simulink library "fixpt_dtprop"  (Simulink 5.0)
undefined symbols (not defined in the file or in its folder): Bias1, Bias2, NumBits1, NumBits2, PosRange1, PosRange2, Slope1, Slope2
libraries: fixpt3 x29, fixpt_lib_4 x1
settings Model: Creator=andyb  LastModifiedBy=kgondoly  ExtModeAutoUpdateStatusClock=off

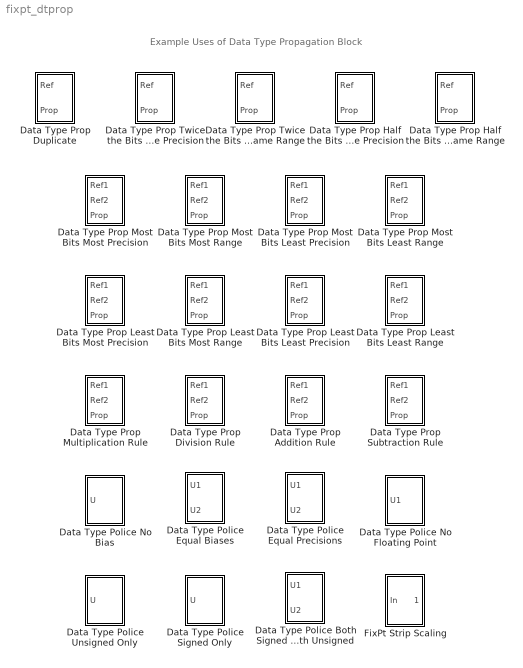
== system fixpt_dtprop ==
  note: Example Uses of Data Type Propagation Block
  Data Type Police Both Signed or Both Unsigned : Subsystem
  Data Type Police Equal Biases : Subsystem
  Data Type Police Equal Precisions : Subsystem
  Data Type Police No Bias : Subsystem
  Data Type Police No Floating Point : Subsystem
  Data Type Police Signed Only : Subsystem
  Data Type Police Unsigned Only : Subsystem
  Data Type Prop Addition Rule : Subsystem
  Data Type Prop Division Rule : Subsystem
  Data Type Prop Duplicate : Subsystem
  Data Type Prop Half the Bits Same Precision : Subsystem
  Data Type Prop Half the Bits Same Range : Subsystem
  Data Type Prop Least Bits Least Precision : Subsystem
  Data Type Prop Least Bits Least Range : Subsystem
  Data Type Prop Least Bits Most Precision : Subsystem
  Data Type Prop Least Bits Most Range : Subsystem
  Data Type Prop Most Bits Least Precision : Subsystem
  Data Type Prop Most Bits Least Range : Subsystem
  Data Type Prop Most Bits Most Precision : Subsystem
  Data Type Prop Most Bits Most Range : Subsystem
  Data Type Prop Multiplication Rule : Subsystem
  Data Type Prop Subtraction Rule : Subsystem
  Data Type Prop Twice the Bits Same Precision : Subsystem
  Data Type Prop Twice the Bits Same Range : Subsystem
  FixPt Strip Scaling : Subsystem
      mask Type: Fixed-Point Strip Scaling
      mask Description: This block strips the scaling off a fixed point signal.  It maps the input data type to the smallest builtin data type that has sufficient bits to hold the input.  The stored Integer Value of the input will be the value of the output.  The output always has nominal scaling (slope = 1.0 and bias = 0.0), so the output does not have a distinction between Real World Value and Stored Integer Value.
      mask Display: fprintf('Strip')

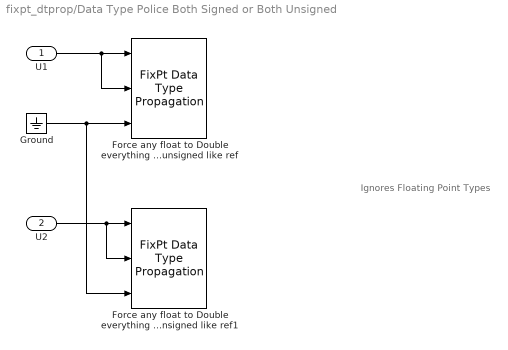
== system fixpt_dtprop/Data Type Police Both Signed or Both Unsigned ==
  note: Ignores Floating Point Types
  U1 : Inport
  U2 : Inport  Port=2
  Force any float to Double everything else to 8 bits with nominal scaling but signed or unsigned like ref : fixpt3/FixPt Data Type Propagation  PropDataType=ufix(8)  IfRefDouble=double  IfRefSingle=double  IsSigned=IsSigned1  NumBitsBase=NumBits1  NumBitsMult=0  NumBitsAdd=8  NumBitsAllowFinal=1:128  PropScalingMode=Specify via dialog  PropScaling=1  SlopeBase=Slope1  SlopeMult=0  SlopeAdd=1  BiasBase=Bias1  BiasMult=1  BiasAdd=0
  Force any float to Double everything else to 8 bits with nominal scaling but signed or unsigned like ref1 : fixpt3/FixPt Data Type Propagation  PropDataType=ufix(8)  IfRefDouble=double  IfRefSingle=double  IsSigned=IsSigned1  NumBitsBase=NumBits1  NumBitsMult=0  NumBitsAdd=8  NumBitsAllowFinal=1:128  PropScalingMode=Specify via dialog  PropScaling=1  SlopeBase=Slope1  SlopeMult=0  SlopeAdd=1  BiasBase=Bias1  BiasMult=1  BiasAdd=0
  Ground : Ground
  wires:
  U1/1 -> Force any float to Double everything else to 8 bits with nominal scaling but signed or unsigned like ref/1, Force any float to Double everything else to 8 bits with nominal scaling but signed or unsigned like ref/2
  Ground/1 -> Force any float to Double everything else to 8 bits with nominal scaling but signed or unsigned like ref1/3, Force any float to Double everything else to 8 bits with nominal scaling but signed or unsigned like ref/3
  U2/1 -> Force any float to Double everything else to 8 bits with nominal scaling but signed or unsigned like ref1/2, Force any float to Double everything else to 8 bits with nominal scaling but signed or unsigned like ref1/1

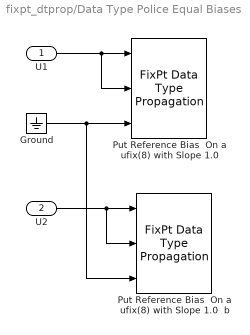
== system fixpt_dtprop/Data Type Police Equal Biases ==
  U1 : Inport
  U2 : Inport  Port=2
  Ground : Ground
  Put Reference Bias  On a ufix(8) with Slope 1.0 : fixpt3/FixPt Data Type Propagation  PropDataTypeMode=Specify via dialog  PropDataType=ufix(8)  IfRefDouble=double  IfRefSingle=double  IsSigned=IsSigned1  NumBitsBase=NumBits1  NumBitsMult=1  NumBitsAdd=0  NumBitsAllowFinal=1:128  PropScaling=2^-10  SlopeBase=Slope1  SlopeMult=0  SlopeAdd=1  BiasBase=Bias1  BiasMult=1  BiasAdd=0
  Put Reference Bias  On a ufix(8) with Slope 1.0  b : fixpt3/FixPt Data Type Propagation  PropDataTypeMode=Specify via dialog  PropDataType=ufix(8)  IfRefDouble=double  IfRefSingle=double  IsSigned=IsSigned1  NumBitsBase=NumBits1  NumBitsMult=1  NumBitsAdd=0  NumBitsAllowFinal=1:128  PropScaling=2^-10  SlopeBase=Slope1  SlopeMult=0  SlopeAdd=1  BiasBase=Bias1  BiasMult=1  BiasAdd=0
  wires:
  U1/1 -> Put Reference Bias  On a ufix(8) with Slope 1.0/2, Put Reference Bias  On a ufix(8) with Slope 1.0/1
  Ground/1 -> Put Reference Bias  On a ufix(8) with Slope 1.0  b/3, Put Reference Bias  On a ufix(8) with Slope 1.0/3
  U2/1 -> Put Reference Bias  On a ufix(8) with Slope 1.0  b/2, Put Reference Bias  On a ufix(8) with Slope 1.0  b/1

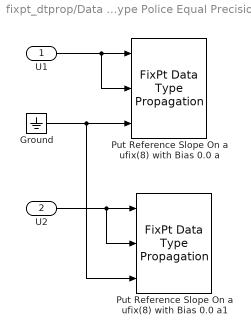
== system fixpt_dtprop/Data Type Police Equal Precisions ==
  U1 : Inport
  U2 : Inport  Port=2
  Ground : Ground
  Put Reference Slope On a ufix(8) with Bias 0.0 a : fixpt3/FixPt Data Type Propagation  PropDataTypeMode=Specify via dialog  PropDataType=ufix(8)  IfRefDouble=double  IfRefSingle=double  IsSigned=IsSigned1  NumBitsBase=NumBits1  NumBitsMult=1  NumBitsAdd=0  NumBitsAllowFinal=1:128  PropScaling=2^-10  SlopeBase=Slope1  SlopeMult=1  SlopeAdd=0  BiasBase=Bias1  BiasMult=0  BiasAdd=0
  Put Reference Slope On a ufix(8) with Bias 0.0 a1 : fixpt3/FixPt Data Type Propagation  PropDataTypeMode=Specify via dialog  PropDataType=ufix(8)  IfRefDouble=double  IfRefSingle=double  IsSigned=IsSigned1  NumBitsBase=NumBits1  NumBitsMult=1  NumBitsAdd=0  NumBitsAllowFinal=1:128  PropScaling=2^-10  SlopeBase=Slope1  SlopeMult=1  SlopeAdd=0  BiasBase=Bias1  BiasMult=0  BiasAdd=0
  wires:
  U2/1 -> Put Reference Slope On a ufix(8) with Bias 0.0 a1/1, Put Reference Slope On a ufix(8) with Bias 0.0 a1/2
  Ground/1 -> Put Reference Slope On a ufix(8) with Bias 0.0 a/3, Put Reference Slope On a ufix(8) with Bias 0.0 a1/3
  U1/1 -> Put Reference Slope On a ufix(8) with Bias 0.0 a/1, Put Reference Slope On a ufix(8) with Bias 0.0 a/2

== system fixpt_dtprop/Data Type Police No Bias ==
  U : Inport
  FixPt Data Type Propagation : fixpt3/FixPt Data Type Propagation  PropDataType=sfix(16)  IfRefDouble=double  IfRefSingle=single  IsSigned=IsSigned1  NumBitsBase=NumBits1  NumBitsMult=1  NumBitsAdd=0  NumBitsAllowFinal=1:128  PropScaling=2^-10  SlopeBase=Slope1  SlopeMult=1  SlopeAdd=0  BiasBase=Bias1  BiasMult=0  BiasAdd=0
  wires:
  U/1 -> FixPt Data Type Propagation/3, FixPt Data Type Propagation/2, FixPt Data Type Propagation/1

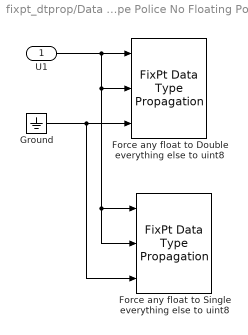
== system fixpt_dtprop/Data Type Police No Floating Point ==
  U1 : Inport
  Force any float to Double everything else to uint8 : fixpt3/FixPt Data Type Propagation  PropDataType=ufix(8)  IfRefDouble=double  IfRefSingle=double  IsSigned=FALSE  NumBitsBase=NumBits1  NumBitsMult=0  NumBitsAdd=8  NumBitsAllowFinal=1:128  PropScalingMode=Specify via dialog  PropScaling=1  SlopeBase=Slope1  SlopeMult=0  SlopeAdd=1  BiasBase=Bias1  BiasMult=1  BiasAdd=0
  Force any float to Single everything else to uint8 : fixpt3/FixPt Data Type Propagation  PropDataType=ufix(8)  IfRefDouble=single  IfRefSingle=single  IsSigned=FALSE  NumBitsBase=NumBits1  NumBitsMult=0  NumBitsAdd=8  NumBitsAllowFinal=1:128  PropScalingMode=Specify via dialog  PropScaling=1  SlopeBase=Slope1  SlopeMult=0  SlopeAdd=1  BiasBase=Bias1  BiasMult=1  BiasAdd=0
  Ground : Ground
  wires:
  Ground/1 -> Force any float to Double everything else to uint8/3, Force any float to Single everything else to uint8/3
  U1/1 -> Force any float to Double everything else to uint8/1, Force any float to Double everything else to uint8/2, Force any float to Single everything else to uint8/2, Force any float to Single everything else to uint8/1

== system fixpt_dtprop/Data Type Police Signed Only ==
  note: Ignores Floating Point Types
  U : Inport
  FixPt Data Type Propagation : fixpt3/FixPt Data Type Propagation  PropDataType=ufix(8)  IfRefDouble=double  IfRefSingle=single  IsSigned=TRUE  NumBitsBase=NumBits1  NumBitsMult=1  NumBitsAdd=0  NumBitsAllowFinal=1:128  PropScaling=1  SlopeBase=Slope1  SlopeMult=1  SlopeAdd=0  BiasBase=Bias1  BiasMult=1  BiasAdd=0
  wires:
  U/1 -> FixPt Data Type Propagation/3, FixPt Data Type Propagation/2, FixPt Data Type Propagation/1

== system fixpt_dtprop/Data Type Police Unsigned Only ==
  note: Ignores Floating Point Types
  U : Inport
  FixPt Data Type Propagation : fixpt3/FixPt Data Type Propagation  PropDataType=ufix(8)  IfRefDouble=double  IfRefSingle=single  IsSigned=FALSE  NumBitsBase=NumBits1  NumBitsMult=1  NumBitsAdd=0  NumBitsAllowFinal=1:128  PropScaling=1  SlopeBase=Slope1  SlopeMult=1  SlopeAdd=0  BiasBase=Bias1  BiasMult=1  BiasAdd=0
  wires:
  U/1 -> FixPt Data Type Propagation/1, FixPt Data Type Propagation/2, FixPt Data Type Propagation/3

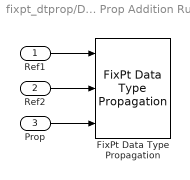
== system fixpt_dtprop/Data Type Prop Addition Rule ==
  Ref1 : Inport
  Ref2 : Inport  Port=2
  Prop : Inport  Port=3
  FixPt Data Type Propagation : fixpt3/FixPt Data Type Propagation  PropDataType=sfix(16)  IfRefDouble=double  IfRefSingle=single  IsSigned=IsSigned1 or IsSigned2  NumBitsBase=max([NumBits1 NumBits2])  NumBitsMult=1  NumBitsAdd=0  NumBitsAllowFinal=1:128  PropScaling=2^-10  SlopeBase=max([PosRange1 PosRange2])  SlopeMult=1  SlopeAdd=0  BiasBase=Bias1+Bias2  BiasMult=1  BiasAdd=0
  wires:
  Ref2/1 -> FixPt Data Type Propagation/2
  Ref1/1 -> FixPt Data Type Propagation/1
  Prop/1 -> FixPt Data Type Propagation/3

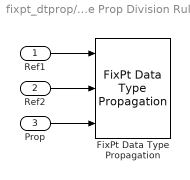
== system fixpt_dtprop/Data Type Prop Division Rule ==
  Ref1 : Inport
  Ref2 : Inport  Port=2
  Prop : Inport  Port=3
  FixPt Data Type Propagation : fixpt3/FixPt Data Type Propagation  PropDataType=sfix(16)  IfRefDouble=double  IfRefSingle=single  IsSigned=IsSigned1 or IsSigned2  NumBitsBase=max([NumBits1 NumBits2])  NumBitsMult=1  NumBitsAdd=0  NumBitsAllowFinal=1:128  PropScaling=2^-10  SlopeBase=Slope1/Slope2  SlopeMult=1  SlopeAdd=0  BiasBase=Bias1/Bias2  BiasMult=1  BiasAdd=0
  wires:
  Prop/1 -> FixPt Data Type Propagation/3
  Ref1/1 -> FixPt Data Type Propagation/1
  Ref2/1 -> FixPt Data Type Propagation/2

== system fixpt_dtprop/Data Type Prop Duplicate ==
  Ref : Inport
  Prop : Inport  Port=2
  FixPt Data Type Propagation : fixpt3/FixPt Data Type Propagation  PropDataType=sfix(16)  IfRefDouble=double  IfRefSingle=single  IsSigned=IsSigned1  NumBitsBase=NumBits1  NumBitsMult=1  NumBitsAdd=0  NumBitsAllowFinal=1:128  PropScaling=2^-10  SlopeBase=Slope1  SlopeMult=1  SlopeAdd=0  BiasBase=Bias1  BiasMult=1  BiasAdd=0
  wires:
  Prop/1 -> FixPt Data Type Propagation/3
  Ref/1 -> FixPt Data Type Propagation/2, FixPt Data Type Propagation/1

== system fixpt_dtprop/Data Type Prop Half the Bits Same Precision ==
  Ref : Inport
  Prop : Inport  Port=2
  FixPt Data Type Propagation : fixpt3/FixPt Data Type Propagation  PropDataType=sfix(16)  IfRefDouble=single  IfRefSingle=single  IsSigned=IsSigned1  NumBitsBase=NumBits1  NumBitsMult=0.5  NumBitsAdd=0  NumBitsAllowFinal=1:128  PropScaling=2^-10  SlopeBase=Slope1  SlopeMult=1  SlopeAdd=0  BiasBase=Bias1  BiasMult=1  BiasAdd=0
  wires:
  Prop/1 -> FixPt Data Type Propagation/3
  Ref/1 -> FixPt Data Type Propagation/2, FixPt Data Type Propagation/1

== system fixpt_dtprop/Data Type Prop Half the Bits Same Range ==
  Ref : Inport
  Prop : Inport  Port=2
  FixPt Data Type Propagation : fixpt3/FixPt Data Type Propagation  PropDataType=sfix(16)  IfRefDouble=single  IfRefSingle=single  IsSigned=IsSigned1  NumBitsBase=NumBits1  NumBitsMult=0.5  NumBitsAdd=0  NumBitsAllowFinal=1:128  PropScaling=2^-10  SlopeBase=PosRange1  SlopeMult=1  SlopeAdd=0  BiasBase=Bias1  BiasMult=1  BiasAdd=0
  wires:
  Ref/1 -> FixPt Data Type Propagation/1, FixPt Data Type Propagation/2
  Prop/1 -> FixPt Data Type Propagation/3

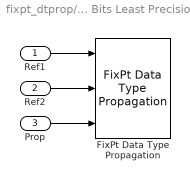
== system fixpt_dtprop/Data Type Prop Least Bits Least Precision ==
  Ref1 : Inport
  Ref2 : Inport  Port=2
  Prop : Inport  Port=3
  FixPt Data Type Propagation : fixpt3/FixPt Data Type Propagation  PropDataType=sfix(16)  IfRefDouble=double  IfRefSingle=single  IsSigned=IsSigned1 or IsSigned2  NumBitsBase=min([NumBits1 NumBits2])  NumBitsMult=1  NumBitsAdd=0  NumBitsAllowFinal=1:128  PropScaling=2^-10  SlopeBase=max([Slope1 Slope2])  SlopeMult=1  SlopeAdd=0  BiasBase=max([Bias1 Bias2])  BiasMult=1  BiasAdd=0
  wires:
  Ref2/1 -> FixPt Data Type Propagation/2
  Ref1/1 -> FixPt Data Type Propagation/1
  Prop/1 -> FixPt Data Type Propagation/3

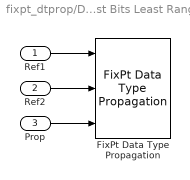
== system fixpt_dtprop/Data Type Prop Least Bits Least Range ==
  Ref1 : Inport
  Ref2 : Inport  Port=2
  Prop : Inport  Port=3
  FixPt Data Type Propagation : fixpt3/FixPt Data Type Propagation  PropDataType=sfix(16)  IfRefDouble=double  IfRefSingle=single  IsSigned=IsSigned1 or IsSigned2  NumBitsBase=min([NumBits1 NumBits2])  NumBitsMult=1  NumBitsAdd=0  NumBitsAllowFinal=1:128  PropScaling=2^-10  SlopeBase=min([PosRange1 PosRange2])  SlopeMult=1  SlopeAdd=0  BiasBase=min([Bias1 Bias2])  BiasMult=1  BiasAdd=0
  wires:
  Prop/1 -> FixPt Data Type Propagation/3
  Ref1/1 -> FixPt Data Type Propagation/1
  Ref2/1 -> FixPt Data Type Propagation/2

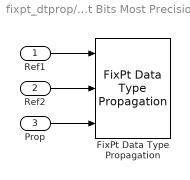
== system fixpt_dtprop/Data Type Prop Least Bits Most Precision ==
  Ref1 : Inport
  Ref2 : Inport  Port=2
  Prop : Inport  Port=3
  FixPt Data Type Propagation : fixpt3/FixPt Data Type Propagation  PropDataType=sfix(16)  IfRefDouble=double  IfRefSingle=single  IsSigned=IsSigned1 or IsSigned2  NumBitsBase=min([NumBits1 NumBits2])  NumBitsMult=1  NumBitsAdd=0  NumBitsAllowFinal=1:128  PropScaling=2^-10  SlopeBase=min([Slope1 Slope2])  SlopeMult=1  SlopeAdd=0  BiasBase=min([Bias1 Bias2])  BiasMult=1  BiasAdd=0
  wires:
  Prop/1 -> FixPt Data Type Propagation/3
  Ref1/1 -> FixPt Data Type Propagation/1
  Ref2/1 -> FixPt Data Type Propagation/2

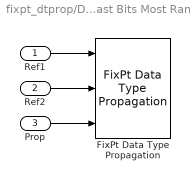
== system fixpt_dtprop/Data Type Prop Least Bits Most Range ==
  Ref1 : Inport
  Ref2 : Inport  Port=2
  Prop : Inport  Port=3
  FixPt Data Type Propagation : fixpt3/FixPt Data Type Propagation  PropDataType=sfix(16)  IfRefDouble=double  IfRefSingle=single  IsSigned=IsSigned1 or IsSigned2  NumBitsBase=min([NumBits1 NumBits2])  NumBitsMult=1  NumBitsAdd=0  NumBitsAllowFinal=1:128  PropScaling=2^-10  SlopeBase=max([PosRange1 PosRange2])  SlopeMult=1  SlopeAdd=0  BiasBase=max([Bias1 Bias2])  BiasMult=1  BiasAdd=0
  wires:
  Ref2/1 -> FixPt Data Type Propagation/2
  Ref1/1 -> FixPt Data Type Propagation/1
  Prop/1 -> FixPt Data Type Propagation/3

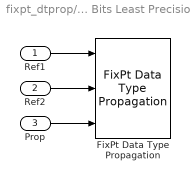
== system fixpt_dtprop/Data Type Prop Most Bits Least Precision ==
  Ref1 : Inport
  Ref2 : Inport  Port=2
  Prop : Inport  Port=3
  FixPt Data Type Propagation : fixpt3/FixPt Data Type Propagation  PropDataType=sfix(16)  IfRefDouble=double  IfRefSingle=single  IsSigned=IsSigned1 or IsSigned2  NumBitsBase=max([NumBits1 NumBits2])  NumBitsMult=1  NumBitsAdd=0  NumBitsAllowFinal=1:128  PropScaling=2^-10  SlopeBase=max([Slope1 Slope2])  SlopeMult=1  SlopeAdd=0  BiasBase=max([Bias1 Bias2])  BiasMult=1  BiasAdd=0
  wires:
  Prop/1 -> FixPt Data Type Propagation/3
  Ref1/1 -> FixPt Data Type Propagation/1
  Ref2/1 -> FixPt Data Type Propagation/2

== system fixpt_dtprop/Data Type Prop Most Bits Least Range ==
  Ref1 : Inport
  Ref2 : Inport  Port=2
  Prop : Inport  Port=3
  FixPt Data Type Propagation : fixpt3/FixPt Data Type Propagation  PropDataType=sfix(16)  IfRefDouble=double  IfRefSingle=single  IsSigned=IsSigned1 or IsSigned2  NumBitsBase=max([NumBits1 NumBits2])  NumBitsMult=1  NumBitsAdd=0  NumBitsAllowFinal=1:128  PropScaling=2^-10  SlopeBase=min([PosRange1 PosRange2])  SlopeMult=1  SlopeAdd=0  BiasBase=min([Bias1 Bias2])  BiasMult=1  BiasAdd=0
  wires:
  Ref2/1 -> FixPt Data Type Propagation/2
  Ref1/1 -> FixPt Data Type Propagation/1
  Prop/1 -> FixPt Data Type Propagation/3

== system fixpt_dtprop/Data Type Prop Most Bits Most Precision ==
  Ref1 : Inport
  Ref2 : Inport  Port=2
  Prop : Inport  Port=3
  FixPt Data Type Propagation : fixpt3/FixPt Data Type Propagation  PropDataType=sfix(16)  IfRefDouble=double  IfRefSingle=single  IsSigned=IsSigned1 or IsSigned2  NumBitsBase=max([NumBits1 NumBits2])  NumBitsMult=1  NumBitsAdd=0  NumBitsAllowFinal=1:128  PropScaling=2^-10  SlopeBase=min([Slope1 Slope2])  SlopeMult=1  SlopeAdd=0  BiasBase=min([Bias1 Bias2])  BiasMult=1  BiasAdd=0
  wires:
  Ref2/1 -> FixPt Data Type Propagation/2
  Ref1/1 -> FixPt Data Type Propagation/1
  Prop/1 -> FixPt Data Type Propagation/3

== system fixpt_dtprop/Data Type Prop Most Bits Most Range ==
  Ref1 : Inport
  Ref2 : Inport  Port=2
  Prop : Inport  Port=3
  FixPt Data Type Propagation : fixpt3/FixPt Data Type Propagation  PropDataType=sfix(16)  IfRefDouble=double  IfRefSingle=single  IsSigned=IsSigned1 or IsSigned2  NumBitsBase=max([NumBits1 NumBits2])  NumBitsMult=1  NumBitsAdd=0  NumBitsAllowFinal=1:128  PropScaling=2^-10  SlopeBase=max([PosRange1 PosRange2])  SlopeMult=1  SlopeAdd=0  BiasBase=max([Bias1 Bias2])  BiasMult=1  BiasAdd=0
  wires:
  Prop/1 -> FixPt Data Type Propagation/3
  Ref1/1 -> FixPt Data Type Propagation/1
  Ref2/1 -> FixPt Data Type Propagation/2

== system fixpt_dtprop/Data Type Prop Multiplication Rule ==
  Ref1 : Inport
  Ref2 : Inport  Port=2
  Prop : Inport  Port=3
  FixPt Data Type Propagation : fixpt3/FixPt Data Type Propagation  PropDataType=sfix(16)  IfRefDouble=double  IfRefSingle=single  IsSigned=IsSigned1 or IsSigned2  NumBitsBase=NumBits1+NumBits2  NumBitsMult=1  NumBitsAdd=0  NumBitsAllowFinal=1:128  PropScaling=2^-10  SlopeBase=Slope1*Slope2  SlopeMult=1  SlopeAdd=0  BiasBase=Bias1*Bias2  BiasMult=1  BiasAdd=0
  wires:
  Ref2/1 -> FixPt Data Type Propagation/2
  Ref1/1 -> FixPt Data Type Propagation/1
  Prop/1 -> FixPt Data Type Propagation/3

== system fixpt_dtprop/Data Type Prop Subtraction Rule ==
  Ref1 : Inport
  Ref2 : Inport  Port=2
  Prop : Inport  Port=3
  FixPt Data Type Propagation : fixpt3/FixPt Data Type Propagation  PropDataType=sfix(16)  IfRefDouble=double  IfRefSingle=single  IsSigned=IsSigned1 or IsSigned2  NumBitsBase=max([NumBits1 NumBits2])  NumBitsMult=1  NumBitsAdd=0  NumBitsAllowFinal=1:128  PropScaling=2^-10  SlopeBase=max([PosRange1 PosRange2])  SlopeMult=1  SlopeAdd=0  BiasBase=Bias1-Bias2  BiasMult=1  BiasAdd=0
  wires:
  Prop/1 -> FixPt Data Type Propagation/3
  Ref1/1 -> FixPt Data Type Propagation/1
  Ref2/1 -> FixPt Data Type Propagation/2

== system fixpt_dtprop/Data Type Prop Twice the Bits Same Precision ==
  Ref : Inport
  Prop : Inport  Port=2
  FixPt Data Type Propagation : fixpt_lib_4/Data Type/Data Type Propagation  PropDataType=sfix(16)  IfRefDouble=double  IfRefSingle=double  IsSigned=IsSigned1  NumBitsBase=NumBits1  NumBitsMult=2  NumBitsAdd=0  NumBitsAllowFinal=1:128  PropScaling=2^-10  ValuesUsedBestPrec=[5 -7]  SlopeBase=Slope1  SlopeMult=1  SlopeAdd=0  BiasBase=Bias1  BiasMult=1  BiasAdd=0
  wires:
  Ref/1 -> FixPt Data Type Propagation/1, FixPt Data Type Propagation/2
  Prop/1 -> FixPt Data Type Propagation/3

== system fixpt_dtprop/Data Type Prop Twice the Bits Same Range ==
  Ref : Inport
  Prop : Inport  Port=2
  FixPt Data Type Propagation : fixpt3/FixPt Data Type Propagation  PropDataType=sfix(16)  IfRefDouble=double  IfRefSingle=double  IsSigned=IsSigned1  NumBitsBase=NumBits1  NumBitsMult=2  NumBitsAdd=0  NumBitsAllowFinal=1:128  PropScaling=2^-10  SlopeBase=PosRange1  SlopeMult=1  SlopeAdd=0  BiasBase=Bias1  BiasMult=1  BiasAdd=0
  wires:
  Prop/1 -> FixPt Data Type Propagation/3
  Ref/1 -> FixPt Data Type Propagation/2, FixPt Data Type Propagation/1

== system fixpt_dtprop/FixPt Strip Scaling ==
  note: Force Scaling to be nominal,
      | slope == 1.0
      | bias == 0.0
  note: Gateway Out set to "auto"
      | which is similar to
      | "Inherit via back propagation"
  In : Inport
  FixPt Data Type Propagation : fixpt3/FixPt Data Type Propagation  PropDataType=sfix(16)  IfRefDouble=double  IfRefSingle=single  IsSigned=IsSigned1  NumBitsBase=NumBits1  NumBitsMult=1  NumBitsAdd=0  NumBitsAllowFinal=[8,16,32]  PropScalingMode=Specify via dialog  PropScaling=1  SlopeBase=Slope1  SlopeMult=0  SlopeAdd=1  BiasBase=Bias1  BiasMult=1  BiasAdd=0
  FixPt Gateway Out : fixpt3/FixPt Gateway Out  OutRealWorld=Stored Integer  OutBuiltInType=auto
  Out1 : Outport
  wires:
  In/1 -> FixPt Data Type Propagation/1, FixPt Data Type Propagation/2, FixPt Gateway Out/1
  FixPt Gateway Out/1 -> FixPt Data Type Propagation/3, Out1/1
